simulink model "Q2_2"  (R2023b)
settings: Solver=VariableStepAuto  StartTime=0.0  StopTime=50  RelTol=1e-3
libraries: mpclib x1, simulink x1
settings Model: Creator=sayed  LastModifiedBy=sayed

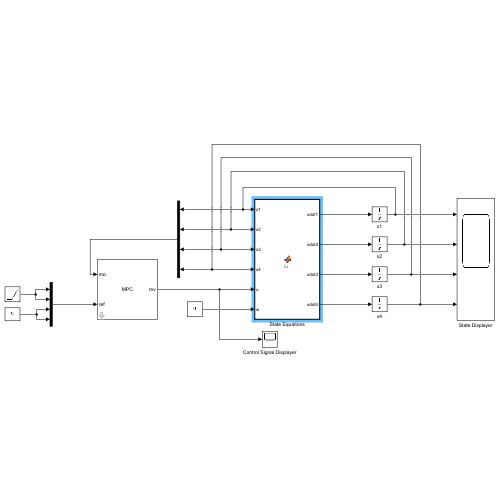
[thumbnail: Simulink's stored preview of the top-level diagram]
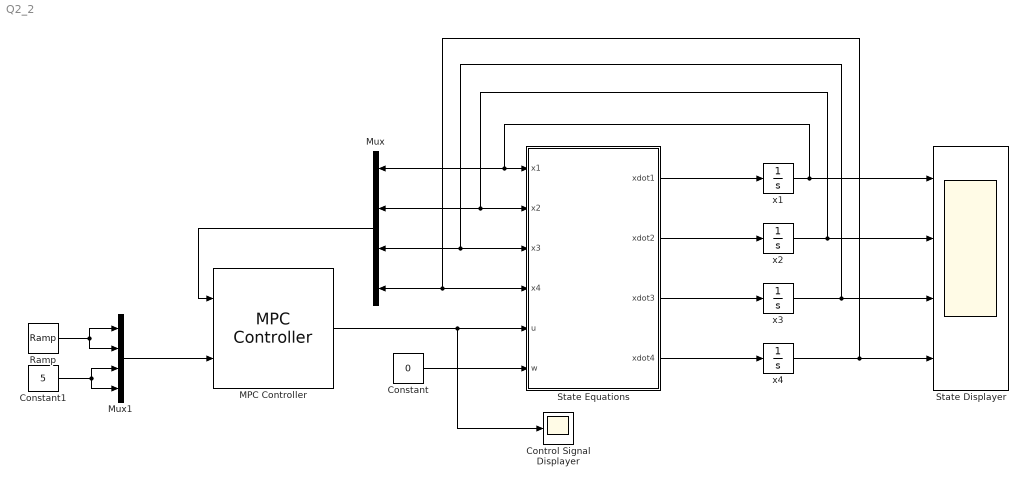
== system Q2_2 ==
  Constant : Constant  Value=0
  Constant1 : Constant  Value=5
  Control Signal Displayer : Scope
  MPC Controller : mpclib/MPC Controller  SCDEnableBlockLinearizationSpecification=on  mpcobj=mpc1  is_multiple=0  enable_value=0  return_u0=off  updateMPCinCallerWorkspace=on  md_inport=off  mv_inport=off  uref_inport=off  return_cost=off  return_mvseq=off  return_qpstatus=off  return_xseq=off  return_state=off  return_ovseq=off  state_inport=off  umin_inport=off  umax_inport=off  ymin_inport=off  ymax_inport=off  cc_inport=off  ywt_inport=off  uwt_inport=off  duwt_inport=off  rhoeps_inport=off  pm_inport=off  MaximumP=10  HorizonChoice=FixedHorizon  n_ts=0.01  n_p=800  n_mv=1  n_md=0  n_ud=0  n_mo=4  n_uo=0  BlockDataType=double  SampleTimeInherited=off  switch_inport=off
  Mux : Mux
  Mux1 : Mux
  Ramp : simulink/Sources/Ramp  slope=5  start=0  InitialOutput=0
  State Displayer : Scope  NumInputPorts=4
  State Equations : MATLAB Function  TreatAsAtomicUnit=on
  x1 : Integrator
  x2 : Integrator
  x3 : Integrator  InitialCondition=2
  x4 : Integrator  InitialCondition=0.5
  wires:
  State Equations/1(xdot1) -> x1/1
  State Equations/2(xdot2) -> x2/1
  State Equations/3(xdot3) -> x3/1
  State Equations/4(xdot4) -> x4/1
  x1/1 -> State Displayer/1, Mux/1, State Equations/1(x1)
  x2/1 -> State Displayer/2, Mux/2, State Equations/2(x2)
  x3/1 -> State Displayer/3, Mux/3, State Equations/3(x3)
  x4/1 -> State Displayer/4, Mux/4, State Equations/4(x4)
  Constant/1 -> State Equations/6(w)
  MPC Controller/1 -> State Equations/5(u), Control Signal Displayer/1
  Ramp/1 -> Mux1/1, Mux1/2
  Mux1/1 -> MPC Controller/2
  Mux/1 -> MPC Controller/1
  Constant1/1 -> Mux1/4, Mux1/3

== matlab function Q2_2/State Equations ==
  data: x1 input; x2 input; x3 input; x4 input; u input; xdot1 output; w input; xdot2 output; xdot3 output; xdot4 output
function [xdot1, xdot2, xdot3, xdot4] = fcn(x1, x2, x3, x4, u, w)

% Parameter Values

m1 = 10000;
m2 = 8000;
k = 500000;
c = 5000;

% State-Equations

xdot1 = x3;
xdot2 = x4;
xdot3 = (1 / m1) * (k * (-x1 + x2) + c * (-x3 + x4) + u + w);
xdot4 = (1 / m2) * (k * (x1 - x2) + c * (x3 - x4));
